simulink model "ESP_Interface"  (R2024a)
settings: Solver=FixedStepAuto  StartTime=0.0  StopTime=10  FixedStep=0.001  RelTol=1e-3  EnableMultiTasking=on
libraries: arduinolib x3, arduinosensorlib x2
settings Model: ExtModeTrigDuration=2  Creator=Ingy  LastModifiedBy=Ingy
settings SolverCC: AutoInsertRateTranBlk=on
settings OptimizationCC: EnhancedBackFolding=on  PassReuseOutputArgsAs=Individual arguments  ZeroExternalMemoryAtStartup=off  ZeroInternalMemoryAtStartup=off  MaxStackSize=64  OptimizeBlockOrder=speed  DifferentSizesBufferReuse=on  OptimizationCustomize=off  EfficientTunableParamExpr=on
settings DebuggingCC: ParameterTunabilityLossMsg=error
settings HardwareCC: ProdBitPerPointer=32  ProdBitPerSizeT=32  ProdBitPerPtrDiffT=32  ProdLargestAtomicInteger=Long  ProdLargestAtomicFloat=Double  ProdWordSize=32  ProdHWDeviceType=ARM Compatible->ARM Cortex  UseEmbeddedCoderFeatures=off
settings SFSimCC: MATLABDynamicMemAlloc=off
settings RTWCC: Description=Embedded Coder  SystemTargetFile=ert.tlc  HardwareBoard=ESP32-WROOM(Arduino Compatible)  TLCOptions="-aInlineSetEventsForThisBaseRateFcn=TLC_FALSE -aSuppressMultiTaskScheduler=TLC_FALSE  -aRateBasedStepFcn=0"  TemplateMakefile=ert_default_tmf  Toolchain=ESP32  BuildConfiguration=Faster Runs
settings CodeAppCC: ForceParamTrailComments=on  IgnoreCustomStorageClasses=off  OperatorAnnotations=on  SimulinkDataObjDesc=on  SFDataObjDesc=on  InsertBlockDesc=on
settings ERTTargetCC: SupportContinuousTime=on  SupportNonInlinedSFcns=on  SupportVariableSizeSignals=on  ExtModeTransport=3  ExtModeStaticAlloc=on  ExtModeAutomaticAllocSize=off  ExtModeStaticAllocSize=65536  ExtModeMexFile=ext_xcp  ExtModeIntrfLevel=Level2 - Open

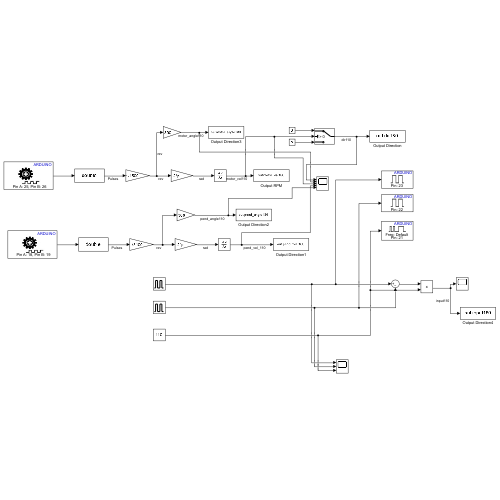
[thumbnail: Simulink's stored preview of the top-level diagram]
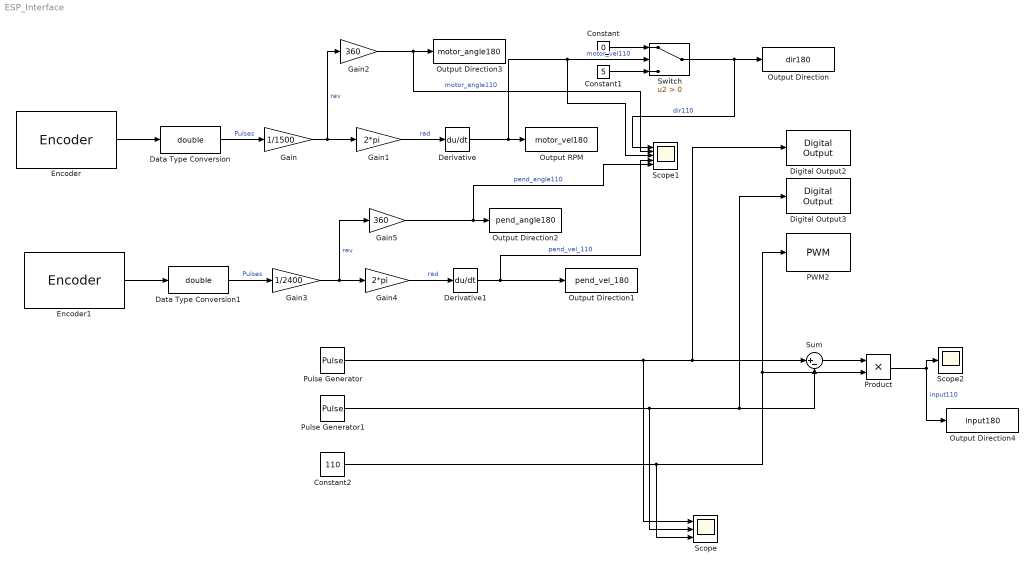
== system ESP_Interface ==
  Constant : Constant  Value=0
  Constant1 : Constant  Value=5
  Constant2 : Constant  Value=110
  Data Type Conversion : DataTypeConversion  OutDataTypeStr=double  SaturateOnIntegerOverflow=off  RndMeth=Floor
  Data Type Conversion1 : DataTypeConversion  OutDataTypeStr=double  SaturateOnIntegerOverflow=off  RndMeth=Floor
  Derivative : Derivative
  Derivative1 : Derivative
  Digital Output2 : arduinolib/Digital Output  pinNumber=23  Direction=output  blockPlatform=arduino
  Digital Output3 : arduinolib/Digital Output  pinNumber=22  Direction=output  blockPlatform=arduino
  Encoder : arduinosensorlib/Encoder  InputA=25  InputB=26  Mode=No reset  SampleTime=-1
  Encoder1 : arduinosensorlib/Encoder  InputA=18  InputB=19  Mode=No reset  SampleTime=-1
  Gain : Gain  Gain=1/1500
  Gain1 : Gain  Gain=2*pi
  Gain2 : Gain  Gain=360
  Gain3 : Gain  Gain=1/2400
  Gain4 : Gain  Gain=2*pi
  Gain5 : Gain  Gain=360
  Output Direction : ToWorkspace  VariableName=dir180  SampleTime=0.01
      settings: Save2DSignal=2-D array (concatenate along first dimension)
  Output Direction1 : ToWorkspace  VariableName=pend_vel_180  SampleTime=0.01
      settings: Save2DSignal=2-D array (concatenate along first dimension)
  Output Direction2 : ToWorkspace  VariableName=pend_angle180  SampleTime=0.01
      settings: Save2DSignal=2-D array (concatenate along first dimension)
  Output Direction3 : ToWorkspace  VariableName=motor_angle180  SampleTime=0.01
      settings: Save2DSignal=2-D array (concatenate along first dimension)
  Output Direction4 : ToWorkspace  VariableName=input180  SampleTime=0.01
      settings: Save2DSignal=2-D array (concatenate along first dimension)
  Output RPM : ToWorkspace  VariableName=motor_vel180  SampleTime=0.01
      settings: Save2DSignal=2-D array (concatenate along first dimension)
  PWM2 : arduinolib/PWM  pinNumber=21  frequencyType=Default  desiredFrequency=490.2  achievableFrequency=490.2
  Product : Product
  Pulse Generator : DiscretePulseGenerator  PulseType=Time based  Period=10  PulseWidth=5  PhaseDelay=1
  Pulse Generator1 : DiscretePulseGenerator  PulseType=Time based  Period=10  PulseWidth=5  PhaseDelay=6
  Scope : Scope  NumInputPorts=3
  Scope1 : Scope  NumInputPorts=5
  Scope2 : Scope
  Sum : Sum  Inputs=|+-
  Switch : Switch  Criteria=u2 > Threshold  SaturateOnIntegerOverflow=off  InputSameDT=off
  wires:
  Switch/1 -> Scope1/1, Output Direction/1  "dir110"
  Constant/1 -> Switch/1
  Gain1/1 -> Derivative/1  "rad"
  Constant1/1 -> Switch/3
  Derivative/1 -> Output RPM/1, Scope1/3, Switch/2  "motor_vel110"
  Data Type Conversion/1 -> Gain/1  "Pulses"
  Encoder/1 -> Data Type Conversion/1
  Gain3/1 -> Gain5/1, Gain4/1  "rev"
  Encoder1/1 -> Data Type Conversion1/1
  Gain4/1 -> Derivative1/1  "rad"
  Derivative1/1 -> Scope1/4, Output Direction1/1  "pend_vel_110"
  Data Type Conversion1/1 -> Gain3/1  "Pulses"
  Gain5/1 -> Scope1/5, Output Direction2/1  "pend_angle110"
  Gain2/1 -> Scope1/2, Output Direction3/1  "motor_angle110"
  Gain/1 -> Gain2/1, Gain1/1  "rev"
  Pulse Generator/1 -> Scope/1, Sum/1, Digital Output2/1
  Constant2/1 -> Scope/3, Product/2, PWM2/1
  Pulse Generator1/1 -> Scope/2, Sum/2, Digital Output3/1
  Sum/1 -> Product/1
  Product/1 -> Scope2/1, Output Direction4/1  "input110"
